simulink model "Katex_FullCar_R2017b_V03"  (R2026a)
settings: Solver=ode1  StopTime=1000  FixedStep=Ts  EnableMultiTasking=on
PostLoadFcn:
  | , if any(exist('dsrtsu_mdlpostloadfcn', 'file') == [2, 3, 6]), try dsrtsu_mdlpostloadfcn('Execute', bdroot); catch fprintf('Error in PostLoadFcn (dsrtsu_mdlpostloadfcn) for model "%s":\n %s\n', bdroot, lasterr); end, end,
  | , if any(exist('dsrtsu_mdlpostloadfcn', 'file') ~= 0), dsrtsu_mdlpostloadfcn('Execute', bdroot); end,
InitFcn:
  | , if any(exist('rtifpga_mdlclblib', 'file') ~= 0), rtifpga_mdlclblib('Init', bdroot); end,
  | 
  | 
  | init
undefined symbols (not defined in the file): locklim_sus, roundN, Ts
libraries: sl_discontinuities x29, simulink_extras x26, simulink x22, mjLib x1
(part 2 of 10)

== system Katex_FullCar_R2017b_V03/Locomotion/Initialization ==
  FLin : Inport
  FRin : Inport  Port=2
  RLin : Inport  Port=3
  RRin : Inport  Port=4
  Bus Creator{1..5} (5 alike) : BusCreator  Inputs=4
  Bus Selector : BusSelector  OutputSignals=FLdrv_velref_mps,FLstr_angref_deg,FLsus_angref_deg
  Bus Selector1 : BusSelector  OutputSignals=FRdrv_velref_mps,FRstr_angref_deg,FRsus_angref_deg
  Bus Selector2 : BusSelector  OutputSignals=RLdrv_velref_mps,RLstr_angref_deg,RLsus_angref_deg
  Bus Selector3 : BusSelector  OutputSignals=RRdrv_velref_mps,RRstr_angref_deg,RRsus_angref_deg
  Subsystem : Subsystem
  Subsystem1 : Subsystem
  Subsystem2 : Subsystem
  Subsystem3 : Subsystem
  Controller : Outport  VectorParamsAs1DForOutWhenUnconnected=off
  tag scope: Controller=global
  wires:
  FLin/1 -> Subsystem/1(In1), Bus Selector/1
  Bus Selector/2 -> Bus Creator4/2  "<FLstr_angref_deg>"
  Bus Selector/3 -> Bus Creator4/3  "<FLsus_angref_deg>"
  Bus Creator4/1 -> Bus Creator5/1  "FL"
  Bus Selector/1 -> Bus Creator4/1  "<FLdrv_velref_mps>"
  FRin/1 -> Subsystem1/1(In1), Bus Selector1/1
  Bus Selector1/1 -> Bus Creator1/1  "<FRdrv_velref_mps>"
  Bus Creator1/1 -> Bus Creator5/2  "FR"
  Bus Creator2/1 -> Bus Creator5/3  "RL"
  RLin/1 -> Subsystem2/1(In1), Bus Selector2/1
  RRin/1 -> Subsystem3/1(In1), Bus Selector3/1
  Bus Creator3/1 -> Bus Creator5/4  "RR"
  Subsystem/1(Out1) -> Bus Creator4/4  "FL_tqctrl"
  Subsystem1/1(Out1) -> Bus Creator1/4  "FR_tqctrl"
  Subsystem2/1(Out1) -> Bus Creator2/4  "RL_tqctrl"
  Subsystem3/1(Out1) -> Bus Creator3/4  "RR_tqctrl"
  Bus Creator5/1 -> [Controller], Controller/1  "Controller"
  Bus Selector1/2 -> Bus Creator1/2  "<FRstr_angref_deg>"
  Bus Selector1/3 -> Bus Creator1/3  "<FRsus_angref_deg>"
  Bus Selector2/1 -> Bus Creator2/1  "<RLdrv_velref_mps>"
  Bus Selector2/2 -> Bus Creator2/2  "<RLstr_angref_deg>"
  Bus Selector2/3 -> Bus Creator2/3  "<RLsus_angref_deg>"
  Bus Selector3/1 -> Bus Creator3/1  "<RRdrv_velref_mps>"
  Bus Selector3/2 -> Bus Creator3/2  "<RRstr_angref_deg>"
  Bus Selector3/3 -> Bus Creator3/3  "<RRsus_angref_deg>"

== system Katex_FullCar_R2017b_V03/MuJoCo Interface/FL_Motor_Control ==
  note: 0: Pos Mode
      | 1: Vel Mode
      | 2: Torque Mode
  In1 : Inport
  Bus Creator1 : BusCreator  Inputs=4
  Constant : Constant  Value=0
  Drv_Driver : Subsystem
  Str_Driver : Subsystem
  Sus_Driver : Subsystem
  Out2 : Outport  VectorParamsAs1DForOutWhenUnconnected=off
  wires:
  [Sus_Driver_Mode] -> Sus_Driver/1(In1)
  In1/1 -> Drv_Driver/2(In2), Str_Driver/2(In2), Sus_Driver/2(In2)
  [Str_Driver_Mode] -> Str_Driver/1(In1)
  [Drv_Driver_Mode] -> Drv_Driver/1(In1)
  Constant/1 -> Bus Creator1/2  "cover_motor"
  Bus Creator1/1 -> Out2/1
  Sus_Driver/1(FL_sus_motor) -> Bus Creator1/1  "FL_sus_act"
  Str_Driver/1(FL_steer_motor) -> Bus Creator1/3  "FL_steer_rev"
  Drv_Driver/1(FL_drive_motor) -> Bus Creator1/4  "FL_drive_act"

== system Katex_FullCar_R2017b_V03/MuJoCo Interface/FR_Motor_Control ==
  note: 0: Pos Mode
      | 1: Vel Mode
      | 2: Torque Mode
  In1 : Inport
  Bus Creator1 : BusCreator  Inputs=4
  Constant : Constant  Value=0
  Drv_Driver : Subsystem
  Str_Driver : Subsystem
  Sus_Driver : Subsystem
  Out2 : Outport  VectorParamsAs1DForOutWhenUnconnected=off
  wires:
  In1/1 -> Sus_Driver/2(In2), Str_Driver/2(In2), Drv_Driver/2(In2)
  Constant/1 -> Bus Creator1/2  "cover_motor"
  Bus Creator1/1 -> Out2/1
  [Sus_Driver_Mode] -> Sus_Driver/1(In1)
  Sus_Driver/1(FR_sus_motor) -> Bus Creator1/1  "FR_sus_act"
  [Str_Driver_Mode] -> Str_Driver/1(In1)
  Str_Driver/1(FR_steer_motor) -> Bus Creator1/3  "FR_steer_rev"
  [Drv_Driver_Mode] -> Drv_Driver/1(In1)
  Drv_Driver/1(FR_drive_motor) -> Bus Creator1/4  "FR_drive_act"

== system Katex_FullCar_R2017b_V03/MuJoCo Interface/RL_Motor_Control ==
  note: 0: Pos Mode
      | 1: Vel Mode
      | 2: Torque Mode
  In1 : Inport
  Bus Creator1 : BusCreator  Inputs=4
  Constant : Constant  Value=0
  Drv_Driver : Subsystem
  Str_Driver : Subsystem
  Sus_Driver : Subsystem
  Out2 : Outport  VectorParamsAs1DForOutWhenUnconnected=off
  wires:
  Bus Creator1/1 -> Out2/1
  Constant/1 -> Bus Creator1/2  "cover_motor"
  In1/1 -> Str_Driver/2(In2), Drv_Driver/2(In2), Sus_Driver/2(In2)
  [Sus_Driver_Mode] -> Sus_Driver/1(In1)
  Sus_Driver/1(RL_sus_motor) -> Bus Creator1/1  "RL_sus_act"
  [Str_Driver_Mode] -> Str_Driver/1(In1)
  Str_Driver/1(RL_steer_motor) -> Bus Creator1/3  "RL_steer_rev"
  [Drv_Driver_Mode] -> Drv_Driver/1(In1)
  Drv_Driver/1(RL_drive_motor) -> Bus Creator1/4  "RL_drive_act"

== system Katex_FullCar_R2017b_V03/MuJoCo Interface/RR_Motor_Control ==
  note: 0: Pos Mode
      | 1: Vel Mode
      | 2: Torque Mode
  In1 : Inport
  Bus Creator1 : BusCreator  Inputs=4
  Constant : Constant  Value=0
  Drv_Driver : Subsystem
  Str_Driver : Subsystem
  Sus_Driver : Subsystem
  Out2 : Outport  VectorParamsAs1DForOutWhenUnconnected=off
  wires:
  In1/1 -> Str_Driver/2(In2), Drv_Driver/2(In2), Sus_Driver/2(In2)
  Constant/1 -> Bus Creator1/2  "cover_motor"
  Bus Creator1/1 -> Out2/1
  [Sus_Driver_Mode] -> Sus_Driver/1(In1)
  Sus_Driver/1(RR_sus_motor) -> Bus Creator1/1  "RR_sus_act"
  [Str_Driver_Mode] -> Str_Driver/1(In1)
  Str_Driver/1(RR_steer_motor) -> Bus Creator1/3  "RR_steer_rev"
  [Drv_Driver_Mode] -> Drv_Driver/1(In1)
  Drv_Driver/1(RR_drive_motor) -> Bus Creator1/4  "RR_drive_act"

== system Katex_FullCar_R2017b_V03/Scope/FL ==
  Plant : Inport
  Controller : Inport  Port=2
  Bus Selector3 : BusSelector  OutputSignals=torque_sensor_FL,ENC_FL_sus,ENC_FL_steer,ENC_FL_drive,Vel_FL_sus,Vel_FL_steer,Vel_FL_drv,FL_sus_actuator_torque
  Bus Selector4 : BusSelector  OutputSignals=FL.FLdrv_velref_mps,FL.FL_tqctrl.FLdrv_tqref_pct,FL.FLstr_angref_deg,FL.FL_tqctrl.FLstr_tqref_pct,FL.FLsus_angref_deg,FL.FL_tqctrl.FLsus_tqref_pct
  Demux : Demux  Outputs=3
  FL_sus_torque : Scope
      settings: ActiveDisplayYMinimum=-1  ActiveDisplayYMaximum=1  DataLoggingVariableName=ScopeData81
  FLdrv_ang[deg] : Scope
      settings: ActiveDisplayYMinimum=-1.4323067935591529  ActiveDisplayYMaximum=1.2660358171832233  DataLoggingVariableName=ScopeData31
  FLdrv_ang[rad] : Scope
      settings: ActiveDisplayYMinimum=-1  ActiveDisplayYMaximum=1  DataLoggingVariableName=ScopeData34
  FLdrv_angvel[rad/s] : Scope
      settings: ActiveDisplayYMinimum=-1  ActiveDisplayYMaximum=1  DataLoggingVariableName=ScopeData68
  FLdrv_torque_x : Scope
      settings: ActiveDisplayYMinimum=-1  ActiveDisplayYMaximum=1  DataLoggingVariableName=ScopeData32
  FLdrv_torque_y : Scope
      settings: ActiveDisplayYMinimum=-1  ActiveDisplayYMaximum=1  DataLoggingVariableName=ScopeData36
  FLdrv_torque_z : Scope
      settings: ActiveDisplayYMinimum=-1  ActiveDisplayYMaximum=1  DataLoggingVariableName=ScopeData29
  FLdrv_tqcmd_pct : Scope
      settings: ActiveDisplayYMinimum=-1  ActiveDisplayYMaximum=1  DataLoggingVariableName=ScopeData33
  FLdrv_tracking_angvel[rad/s] : Scope  NumInputPorts=2
      settings: ActiveDisplayYMinimum=-0.28030249586528166  ActiveDisplayYMaximum=1.28308219274336  DataLoggingVariableName=ScopeData6
  FLdrv_velcmd_mps : Scope
      settings: ActiveDisplayYMinimum=-1  ActiveDisplayYMaximum=1  DataLoggingVariableName=ScopeData35
  FLstr_ang[deg] : Scope
      settings: ActiveDisplayYMinimum=-1  ActiveDisplayYMaximum=1  DataLoggingVariableName=ScopeData22
  FLstr_ang[rad] : Scope
      settings: ActiveDisplayYMinimum=-1  ActiveDisplayYMaximum=1  DataLoggingVariableName=ScopeData38
  FLstr_angcmd_deg : Scope
      settings: ActiveDisplayYMinimum=-1  ActiveDisplayYMaximum=1  DataLoggingVariableName=ScopeData37
  FLstr_angvel[rad/s] : Scope
      settings: ActiveDisplayYMinimum=-1  ActiveDisplayYMaximum=1  DataLoggingVariableName=ScopeData25
  FLstr_tqcmd_pct : Scope
      settings: ActiveDisplayYMinimum=-1  ActiveDisplayYMaximum=1  DataLoggingVariableName=ScopeData40
  FLstr_tracking_ang[deg] : Scope  NumInputPorts=2
      settings: ActiveDisplayYMinimum=-11.551242119792914  ActiveDisplayYMaximum=16.207341064536273
  FLsus_ang[deg] : Scope
      settings: ActiveDisplayYMinimum=-37.299932165417033  ActiveDisplayYMaximum=37.7179622752956  DataLoggingVariableName=ScopeData23
  FLsus_ang[rad] : Scope
      settings: ActiveDisplayYMinimum=-0.24149003314993756  ActiveDisplayYMaximum=2.1734102983494212  DataLoggingVariableName=ScopeData41
  FLsus_angcmd_deg : Scope
      settings: ActiveDisplayYMinimum=-37.5  ActiveDisplayYMaximum=37.5  DataLoggingVariableName=ScopeData42
  FLsus_angvel[rad/s] : Scope
      settings: ActiveDisplayYMinimum=-1  ActiveDisplayYMaximum=1  DataLoggingVariableName=ScopeData24
  FLsus_tqcmd_pct : Scope
      settings: ActiveDisplayYMinimum=-1  ActiveDisplayYMaximum=1  DataLoggingVariableName=ScopeData45
  FLsus_tracking_ang[deg] : Scope  NumInputPorts=2
      settings: ActiveDisplayYMinimum=-59.009615958317596  ActiveDisplayYMaximum=72.033120306985637  DataLoggingVariableName=ScopeData23
  Radians to Degrees : simulink_extras/Transformations/Radians to Degrees
  Radians to Degrees1 : simulink_extras/Transformations/Radians to Degrees
  Radians to Degrees2 : simulink_extras/Transformations/Radians to Degrees
  Subsystem13 : Subsystem
      mask Display: disp('Dri_ref(m/s)_2_motor(rad/s)');
  tag scope: FL_sus_torque=global, FLdrv_ang_deg=global, FLdrv_ang_rad=global, FLdrv_angvel_rads=global, FLstr_ang_deg=global, FLstr_ang_rad=global, FLstr_angvel_rads=global, FLsus_ang_deg=global, FLsus_ang_rad=global, FLsus_angvel_rads=global
  wires:
  Bus Selector4/3 -> FLstr_tracking_ang[deg]/1, FLstr_angcmd_deg/1  "<FLstr_angref_deg>"
  Bus Selector4/2 -> FLdrv_tqcmd_pct/1  "<FLdrv_tqref_pct>"
  Controller/1 -> Bus Selector4/1
  Bus Selector4/5 -> FLsus_tracking_ang[deg]/1, FLsus_angcmd_deg/1  "<FLsus_angref_deg>"
  Bus Selector4/1 -> Subsystem13/1(In1), FLdrv_velcmd_mps/1  "<FLdrv_velref_mps>"
  Bus Selector4/4 -> FLstr_tqcmd_pct/1  "<FLstr_tqref_pct>"
  Bus Selector4/6 -> FLsus_tqcmd_pct/1  "<FLsus_tqref_pct>"
  Plant/1 -> Bus Selector3/1
  Bus Selector3/1 -> Demux/1  "<torque_sensor_FL>"
  Demux/1 -> FLdrv_torque_x/1
  Demux/2 -> FLdrv_torque_y/1
  Demux/3 -> FLdrv_torque_z/1
  Bus Selector3/2 -> [FLsus_ang_rad], Radians to Degrees1/1, FLsus_ang[rad]/1  "<ENC_FL_sus>"
  Bus Selector3/3 -> [FLstr_ang_rad], Radians to Degrees/1, FLstr_ang[rad]/1  "<ENC_FL_steer>"
  Bus Selector3/4 -> [FLdrv_ang_rad], FLdrv_ang[rad]/1, Radians to Degrees2/1  "<ENC_FL_drive>"
  Radians to Degrees/1 -> FLstr_tracking_ang[deg]/2, FLstr_ang[deg]/1, [FLstr_ang_deg]
  Radians to Degrees1/1 -> FLsus_tracking_ang[deg]/2, FLsus_ang[deg]/1, [FLsus_ang_deg]
  Radians to Degrees2/1 -> FLdrv_ang[deg]/1, [FLdrv_ang_deg]
  Bus Selector3/5 -> [FLsus_angvel_rads], FLsus_angvel[rad/s]/1  "<Vel_FL_sus>"
  Bus Selector3/6 -> [FLstr_angvel_rads], FLstr_angvel[rad/s]/1  "<Vel_FL_steer>"
  Bus Selector3/7 -> [FLdrv_angvel_rads], FLdrv_angvel[rad/s]/1  "<Vel_FL_drv>"
  [FLdrv_angvel_rads] -> FLdrv_tracking_angvel[rad/s]/2
  Subsystem13/1(Out1) -> FLdrv_tracking_angvel[rad/s]/1
  Bus Selector3/8 -> FL_sus_torque/1, [FL_sus_torque]  "<FL_sus_actuator_torque>"

== system Katex_FullCar_R2017b_V03/Scope/FR ==
  Plant : Inport
  Controller : Inport  Port=2
  Bus Selector3 : BusSelector  OutputSignals=torque_sensor_FR,ENC_FR_sus,ENC_FR_steer,ENC_FR_drive,Vel_FR_sus,Vel_FR_steer,Vel_FR_drv,FR_sus_actuator_torque
  Bus Selector4 : BusSelector  OutputSignals=FR.FRdrv_velref_mps,FR.FR_tqctrl.FRdrv_tqref_pct,FR.FRstr_angref_deg,FR.FR_tqctrl.FRstr_tqref_pct,FR.FRsus_angref_deg,FR.FR_tqctrl.FRsus_tqref_pct
  Demux : Demux  Outputs=3
  FR_Sus_Torque : Scope
      settings: ActiveDisplayYMinimum=-1  ActiveDisplayYMaximum=1  DataLoggingVariableName=ScopeData93
  FRdrv_ang[deg] : Scope
      settings: ActiveDisplayYMinimum=-1.4323067935591529  ActiveDisplayYMaximum=1.2660358171832233  DataLoggingVariableName=ScopeData26
  FRdrv_ang[rad] : Scope
      settings: ActiveDisplayYMinimum=-0.62767594412282379  ActiveDisplayYMaximum=4.4947333096318136  DataLoggingVariableName=ScopeData30
  FRdrv_angvel[rad/s] : Scope
      settings: ActiveDisplayYMinimum=-1  ActiveDisplayYMaximum=1  DataLoggingVariableName=ScopeData69
  FRdrv_torque_x : Scope
      settings: DataLoggingVariableName=ScopeData39
  FRdrv_torque_y : Scope
      settings: DataLoggingVariableName=ScopeData43
  FRdrv_torque_z : Scope
      settings: DataLoggingVariableName=ScopeData44
  FRdrv_tqcmd_pct : Scope
      settings: DataLoggingVariableName=ScopeData16
  FRdrv_velcmd_mps : Scope
      settings: ActiveDisplayYMinimum=-0.05625  ActiveDisplayYMaximum=0.0062499999999999986  DataLoggingVariableName=ScopeData17
  FRstr_ang[deg] : Scope
      settings: ActiveDisplayYMinimum=-0.68942300067389928  ActiveDisplayYMaximum=1.3010314169983053  DataLoggingVariableName=ScopeData46
  FRstr_ang[rad] : Scope
      settings: ActiveDisplayYMinimum=-1.4323067935591529  ActiveDisplayYMaximum=1.2660358171832233  DataLoggingVariableName=ScopeData47
  FRstr_angcmd_deg : Scope
      settings: ActiveDisplayYMinimum=-1  ActiveDisplayYMaximum=1  DataLoggingVariableName=ScopeData18
  FRstr_angvel[rad/s] : Scope
      settings: ActiveDisplayYMinimum=-1  ActiveDisplayYMaximum=1  DataLoggingVariableName=ScopeData70
  FRstr_tqcmd_pct : Scope
      settings: ActiveDisplayYMinimum=-1  ActiveDisplayYMaximum=1  DataLoggingVariableName=ScopeData19
  FRsus_ang[deg] : Scope
      settings: ActiveDisplayYMinimum=-1.4323067935591529  ActiveDisplayYMaximum=1.2660358171832233  DataLoggingVariableName=ScopeData48
  FRsus_ang[rad] : Scope
      settings: ActiveDisplayYMinimum=-0.24149003314993756  ActiveDisplayYMaximum=2.1734102983494212  DataLoggingVariableName=ScopeData49
  FRsus_angcmd_deg : Scope
      settings: ActiveDisplayYMinimum=-0.15656346548746433  ActiveDisplayYMaximum=1.4090711893871792  DataLoggingVariableName=ScopeData20
  FRsus_angvel[rad/s] : Scope
      settings: ActiveDisplayYMinimum=-1  ActiveDisplayYMaximum=1  DataLoggingVariableName=ScopeData71
  FRsus_tqcmd_pct : Scope
      settings: ActiveDisplayYMinimum=-1  ActiveDisplayYMaximum=1  DataLoggingVariableName=ScopeData21
  Radians to Degrees2 : simulink_extras/Transformations/Radians to Degrees
  Radians to Degrees3 : simulink_extras/Transformations/Radians to Degrees
  Radians to Degrees4 : simulink_extras/Transformations/Radians to Degrees
  tag scope: FR_sus_torque=global, FRdrv_ang_deg=global, FRdrv_ang_rad=global, FRdrv_angvel_rads=global, FRstr_ang_deg=global, FRstr_ang_rad=global, FRstr_angvel_rads=global, FRsus_ang_deg=global, FRsus_ang_rad=global, FRsus_angvel_rads=global
  wires:
  Bus Selector4/3 -> FRstr_angcmd_deg/1  "<FRstr_angref_deg>"
  Bus Selector4/4 -> FRstr_tqcmd_pct/1  "<FRstr_tqref_pct>"
  Bus Selector4/1 -> FRdrv_velcmd_mps/1  "<FRdrv_velref_mps>"
  Bus Selector4/2 -> FRdrv_tqcmd_pct/1  "<FRdrv_tqref_pct>"
  Bus Selector4/5 -> FRsus_angcmd_deg/1  "<FRsus_angref_deg>"
  Bus Selector4/6 -> FRsus_tqcmd_pct/1  "<FRsus_tqref_pct>"
  Demux/2 -> FRdrv_torque_y/1
  Bus Selector3/1 -> Demux/1  "<torque_sensor_FR>"
  Radians to Degrees2/1 -> FRstr_ang[deg]/1, [FRstr_ang_deg]
  Demux/1 -> FRdrv_torque_x/1
  Demux/3 -> FRdrv_torque_z/1
  Bus Selector3/4 -> Radians to Degrees4/1, FRdrv_ang[rad]/1, [FRdrv_ang_rad]  "<ENC_FR_drive>"
  Radians to Degrees4/1 -> FRdrv_ang[deg]/1, [FRdrv_ang_deg]
  Bus Selector3/3 -> Radians to Degrees2/1, FRstr_ang[rad]/1, [FRstr_ang_rad]  "<ENC_FR_steer>"
  Radians to Degrees3/1 -> FRsus_ang[deg]/1, [FRsus_ang_deg]
  Bus Selector3/2 -> [FRsus_ang_rad], Radians to Degrees3/1, FRsus_ang[rad]/1  "<ENC_FR_sus>"
  Controller/1 -> Bus Selector4/1
  Plant/1 -> Bus Selector3/1
  Bus Selector3/6 -> FRstr_angvel[rad/s]/1, [FRstr_angvel_rads]  "<Vel_FR_steer>"
  Bus Selector3/7 -> FRdrv_angvel[rad/s]/1, [FRdrv_angvel_rads]  "<Vel_FR_drv>"
  Bus Selector3/5 -> FRsus_angvel[rad/s]/1, [FRsus_angvel_rads]  "<Vel_FR_sus>"
  Bus Selector3/8 -> [FR_sus_torque], FR_Sus_Torque/1  "<FR_sus_actuator_torque>"

== system Katex_FullCar_R2017b_V03/Scope/IMU ==
  In1 : Inport
  AccX_mps2 : Scope
  AccY_mps2 : Scope
      settings: DataLoggingVariableName=ScopeData2
  AccZ_mps2 : Scope
      settings: DataLoggingVariableName=ScopeData3
  AngPitch_deg : Scope
      settings: ActiveDisplayYMinimum=-1.4665013173998793  ActiveDisplayYMaximum=0.16294459082234145  DataLoggingVariableName=ScopeData8
  AngRoll_deg : Scope
      settings: ActiveDisplayYMinimum=-0.015240922681418762  ActiveDisplayYMaximum=0.083964012205553593  DataLoggingVariableName=ScopeData7
  AngYaw_deg : Scope
      settings: ActiveDisplayYMinimum=-23.87219812859848  ActiveDisplayYMaximum=3.7709983036777981  DataLoggingVariableName=ScopeData15
  Bus Selector : BusSelector  OutputSignals=imu_acc,imu_gyro,trunk_ang
  Demux : Demux  Outputs=3
  Demux1 : Demux  Outputs=3
  Demux2 : Demux  Outputs=3
  Gain1 : Gain
  MATLAB Function : MATLAB Function  TreatAsAtomicUnit=on
  Quaternions to Rotation Angles : Quat2Angle
      settings: AttributesFormatString=Rotation Order: %<rotationOrder>
  Radians to Degrees{,1..5} (6 alike) : simulink_extras/Transformations/Radians to Degrees
  RatePitch_degps : Scope
      settings: DataLoggingVariableName=ScopeData5
  RateRoll_degps : Scope
      settings: DataLoggingVariableName=ScopeData4
  RateYaw_degps : Scope
      settings: DataLoggingVariableName=ScopeData6
  sensor : Gain
  tag scope: AngPitch_deg=global, AngRateYaw_degps=global, AngRoll_deg=global
  wires:
  In1/1 -> Bus Selector/1
  Demux/1 -> AccX_mps2/1
  Demux/2 -> AccY_mps2/1
  Demux/3 -> AccZ_mps2/1
  Bus Selector/1 -> Demux/1  "<imu_acc>"
  Demux1/1 -> Radians to Degrees3/1
  Demux1/2 -> Radians to Degrees4/1
  Demux1/3 -> Radians to Degrees5/1
  Bus Selector/2 -> Demux1/1  "<imu_gyro>"
  Bus Selector/3 -> MATLAB Function/1(q_in)  "<trunk_ang>"
  Quaternions to Rotation Angles/1 -> Demux2/1
  Demux2/2 -> Radians to Degrees1/1
  Demux2/1 -> Radians to Degrees/1
  Demux2/3 -> Radians to Degrees2/1
  Radians to Degrees/1 -> sensor/1
  Radians to Degrees1/1 -> Gain1/1
  Radians to Degrees2/1 -> [AngRoll_deg], AngRoll_deg/1
  Radians to Degrees3/1 -> RateRoll_degps/1
  Radians to Degrees4/1 -> RatePitch_degps/1
  Radians to Degrees5/1 -> [AngRateYaw_degps], RateYaw_degps/1
  MATLAB Function/1(qout) -> Quaternions to Rotation Angles/1
  Gain1/1 -> [AngPitch_deg], AngPitch_deg/1
  sensor/1 -> AngYaw_deg/1  "Sensor"

== system Katex_FullCar_R2017b_V03/Scope/Initialization_Status ==
  InitSta_FLstr : Scope
      settings: ActiveDisplayYMinimum=-1  ActiveDisplayYMaximum=1
  InitSta_FLsus : Scope
      settings: ActiveDisplayYMinimum=-1  ActiveDisplayYMaximum=1  DataLoggingVariableName=ScopeData2
  InitSta_FRstr : Scope
      settings: DataLoggingVariableName=ScopeData8
  InitSta_FRsus : Scope
      settings: DataLoggingVariableName=ScopeData9
  InitSta_RLstr : Scope
      settings: DataLoggingVariableName=ScopeData10
  InitSta_RLsus : Scope
      settings: DataLoggingVariableName=ScopeData11
  InitSta_RRstr : Scope
      settings: DataLoggingVariableName=ScopeData12
  InitSta_RRsus : Scope
      settings: DataLoggingVariableName=ScopeData13
  wires:
  [InitSta_FLstr] -> InitSta_FLstr/1
  [InitSta_FLsus] -> InitSta_FLsus/1
  [InitSta_FRstr] -> InitSta_FRstr/1
  [InitSta_FRsus] -> InitSta_FRsus/1
  [InitSta_RLstr] -> InitSta_RLstr/1
  [InitSta_RLsus] -> InitSta_RLsus/1
  [InitSta_RRstr] -> InitSta_RRstr/1
  [InitSta_RRsus] -> InitSta_RRsus/1

== system Katex_FullCar_R2017b_V03/Scope/RL ==
  Plant : Inport
  Controller : Inport  Port=2
  Bus Selector3 : BusSelector  OutputSignals=torque_sensor_RL,ENC_RL_sus,ENC_RL_steer,ENC_RL_drive,Vel_RL_sus,Vel_RL_steer,Vel_RL_drv,RL_sus_actuator_torque
  Bus Selector4 : BusSelector  OutputSignals=RL.RLdrv_velref_mps,RL.RL_tqctrl.RLdrv_tqref_pct,RL.RLstr_angref_deg,RL.RL_tqctrl.RLstr_tqref_pct,RL.RLsus_angref_deg,RL.RL_tqctrl.RLsus_tqref_pct
  Demux : Demux  Outputs=3
  RL_sus_torque : Scope
      settings: ActiveDisplayYMinimum=-1  ActiveDisplayYMaximum=1  DataLoggingVariableName=ScopeData94
  RLdrv_ang[deg] : Scope
      settings: ActiveDisplayYMinimum=-1.4323067935591529  ActiveDisplayYMaximum=1.2660358171832233  DataLoggingVariableName=ScopeData50
  RLdrv_ang[rad] : Scope
      settings: ActiveDisplayYMinimum=-0.62767594412282379  ActiveDisplayYMaximum=4.4947333096318136  DataLoggingVariableName=ScopeData51
  RLdrv_angvel[rad/s] : Scope
      settings: ActiveDisplayYMinimum=-1  ActiveDisplayYMaximum=1  DataLoggingVariableName=ScopeData72
  RLdrv_torque_x : Scope
      settings: DataLoggingVariableName=ScopeData52
  RLdrv_torque_y : Scope
      settings: DataLoggingVariableName=ScopeData53
  RLdrv_torque_z : Scope
      settings: DataLoggingVariableName=ScopeData54
  RLdrv_tqcmd_pct : Scope
      settings: DataLoggingVariableName=ScopeData33
  RLdrv_velcmd_mps : Scope
      settings: DataLoggingVariableName=ScopeData35
  RLstr_ang[deg] : Scope
      settings: ActiveDisplayYMinimum=-1.4323067935591529  ActiveDisplayYMaximum=1.2660358171832233  DataLoggingVariableName=ScopeData55
  RLstr_ang[rad] : Scope
      settings: ActiveDisplayYMinimum=-1.4323067935591529  ActiveDisplayYMaximum=1.2660358171832233  DataLoggingVariableName=ScopeData56
  RLstr_angcmd_deg : Scope
      settings: DataLoggingVariableName=ScopeData37
  RLstr_angvel[rad/s] : Scope
      settings: ActiveDisplayYMinimum=-1  ActiveDisplayYMaximum=1  DataLoggingVariableName=ScopeData73
  RLstr_tqcmd_pct : Scope
      settings: DataLoggingVariableName=ScopeData40
  RLsus_ang[deg] : Scope
      settings: ActiveDisplayYMinimum=-1.4323067935591529  ActiveDisplayYMaximum=1.2660358171832233  DataLoggingVariableName=ScopeData57
  RLsus_ang[rad] : Scope
      settings: ActiveDisplayYMinimum=-0.24149003314993756  ActiveDisplayYMaximum=2.1734102983494212  DataLoggingVariableName=ScopeData58
  RLsus_angcmd_deg : Scope
      settings: DataLoggingVariableName=ScopeData42
  RLsus_angvel[rad/s] : Scope
      settings: ActiveDisplayYMinimum=-1  ActiveDisplayYMaximum=1  DataLoggingVariableName=ScopeData74
  RLsus_tqcmd_pct : Scope
      settings: DataLoggingVariableName=ScopeData45
  Radians to Degrees2 : simulink_extras/Transformations/Radians to Degrees
  Radians to Degrees3 : simulink_extras/Transformations/Radians to Degrees
  Radians to Degrees4 : simulink_extras/Transformations/Radians to Degrees
  tag scope: RL_sus_torque=global, RLdrv_ang_deg=global, RLdrv_ang_rad=global, RLdrv_angvel_rads=global, RLstr_ang_deg=global, RLstr_ang_rad=global, RLstr_angvel_rads=global, RLsus_ang_deg=global, RLsus_ang_rad=global, RLsus_angvel_rads=global
  wires:
  Bus Selector4/3 -> RLstr_angcmd_deg/1  "<RLstr_angref_deg>"
  Bus Selector4/2 -> RLdrv_tqcmd_pct/1  "<RLdrv_tqref_pct>"
  Controller/1 -> Bus Selector4/1
  Bus Selector4/5 -> RLsus_angcmd_deg/1  "<RLsus_angref_deg>"
  Bus Selector4/1 -> RLdrv_velcmd_mps/1  "<RLdrv_velref_mps>"
  Bus Selector4/4 -> RLstr_tqcmd_pct/1  "<RLstr_tqref_pct>"
  Bus Selector4/6 -> RLsus_tqcmd_pct/1  "<RLsus_tqref_pct>"
  Bus Selector3/1 -> Demux/1  "<torque_sensor_RL>"
  Demux/1 -> RLdrv_torque_x/1
  Radians to Degrees2/1 -> RLstr_ang[deg]/1, [RLstr_ang_deg]
  Radians to Degrees3/1 -> RLsus_ang[deg]/1, [RLsus_ang_deg]
  Bus Selector3/2 -> Radians to Degrees3/1, RLsus_ang[rad]/1, [RLsus_ang_rad]  "<ENC_RL_sus>"
  Radians to Degrees4/1 -> RLdrv_ang[deg]/1, [RLdrv_ang_deg]
  Bus Selector3/4 -> Radians to Degrees4/1, RLdrv_ang[rad]/1, [RLdrv_ang_rad]  "<ENC_RL_drive>"
  Bus Selector3/3 -> Radians to Degrees2/1, RLstr_ang[rad]/1, [RLstr_ang_rad]  "<ENC_RL_steer>"
  Demux/2 -> RLdrv_torque_y/1
  Demux/3 -> RLdrv_torque_z/1
  Plant/1 -> Bus Selector3/1
  Bus Selector3/6 -> RLstr_angvel[rad/s]/1, [RLstr_angvel_rads]  "<Vel_RL_steer>"
  Bus Selector3/7 -> RLdrv_angvel[rad/s]/1, [RLdrv_angvel_rads]  "<Vel_RL_drv>"
  Bus Selector3/5 -> RLsus_angvel[rad/s]/1, [RLsus_angvel_rads]  "<Vel_RL_sus>"
  Bus Selector3/8 -> [RL_sus_torque], RL_sus_torque/1  "<RL_sus_actuator_torque>"

== system Katex_FullCar_R2017b_V03/Scope/RR ==
  Plant : Inport
  Controller : Inport  Port=2
  Bus Selector3 : BusSelector  OutputSignals=torque_sensor_RR,ENC_RR_sus,ENC_RR_steer,ENC_RR_drive,Vel_RR_sus,Vel_RR_steer,Vel_RR_drv,RR_sus_actuator_torque
  Bus Selector4 : BusSelector  OutputSignals=RR.RRdrv_velref_mps,RR.RR_tqctrl.RRdrv_tqref_pct,RR.RRstr_angref_deg,RR.RR_tqctrl.RRstr_tqref_pct,RR.RRsus_angref_deg,RR.RR_tqctrl.RRsus_tqref_pct
  Demux : Demux  Outputs=3
  RLdrv_torque_x : Scope
      settings: DataLoggingVariableName=ScopeData61
  RLdrv_torque_y : Scope
      settings: DataLoggingVariableName=ScopeData62
  RLdrv_torque_z : Scope
      settings: DataLoggingVariableName=ScopeData63
  RR_Sus_torque : Scope
      settings: ActiveDisplayYMinimum=-1  ActiveDisplayYMaximum=1  DataLoggingVariableName=ScopeData95
  RRdrv_ang[deg] : Scope
      settings: ActiveDisplayYMinimum=-1.4323067935591529  ActiveDisplayYMaximum=1.2660358171832233  DataLoggingVariableName=ScopeData59
  RRdrv_ang[rad] : Scope
      settings: ActiveDisplayYMinimum=-0.62767594412282379  ActiveDisplayYMaximum=4.4947333096318136  DataLoggingVariableName=ScopeData60
  RRdrv_angvel[rad/s] : Scope
      settings: ActiveDisplayYMinimum=-1  ActiveDisplayYMaximum=1  DataLoggingVariableName=ScopeData75
  RRdrv_tqcmd_pct : Scope
      settings: DataLoggingVariableName=ScopeData33
  RRdrv_velcmd_mps : Scope
      settings: DataLoggingVariableName=ScopeData35
  RRstr_ang[deg] : Scope
      settings: ActiveDisplayYMinimum=-1.4323067935591529  ActiveDisplayYMaximum=1.2660358171832233  DataLoggingVariableName=ScopeData64
  RRstr_ang[rad] : Scope
      settings: ActiveDisplayYMinimum=-1.4323067935591529  ActiveDisplayYMaximum=1.2660358171832233  DataLoggingVariableName=ScopeData65
  RRstr_angcmd_deg : Scope
      settings: DataLoggingVariableName=ScopeData37
  RRstr_angvel[rad/s] : Scope
      settings: ActiveDisplayYMinimum=-1  ActiveDisplayYMaximum=1  DataLoggingVariableName=ScopeData76
  RRstr_tqcmd_pct : Scope
      settings: DataLoggingVariableName=ScopeData40
  RRsus_ang[deg] : Scope
      settings: ActiveDisplayYMinimum=-1.4323067935591529  ActiveDisplayYMaximum=1.2660358171832233  DataLoggingVariableName=ScopeData66
  RRsus_ang[rad] : Scope
      settings: ActiveDisplayYMinimum=-0.24149003314993756  ActiveDisplayYMaximum=2.1734102983494212  DataLoggingVariableName=ScopeData67
  RRsus_angcmd_deg : Scope
      settings: DataLoggingVariableName=ScopeData42
  RRsus_angvel[rad/s] : Scope
      settings: ActiveDisplayYMinimum=-1  ActiveDisplayYMaximum=1  DataLoggingVariableName=ScopeData77
  RRsus_tqcmd_pct : Scope
      settings: DataLoggingVariableName=ScopeData45
  Radians to Degrees2 : simulink_extras/Transformations/Radians to Degrees
  Radians to Degrees3 : simulink_extras/Transformations/Radians to Degrees
  Radians to Degrees4 : simulink_extras/Transformations/Radians to Degrees
  tag scope: RR_Sus_torque=global, RRdrv_ang_deg=global, RRdrv_ang_rad=global, RRdrv_angvel_rads=global, RRstr_ang_deg=global, RRstr_ang_rad=global, RRstr_angvel_rads=global, RRsus_ang_deg=global, RRsus_ang_rad=global, RRsus_angvel_rads=global
  wires:
  Bus Selector4/3 -> RRstr_angcmd_deg/1  "<RRstr_angref_deg>"
  Bus Selector4/2 -> RRdrv_tqcmd_pct/1  "<RRdrv_tqref_pct>"
  Controller/1 -> Bus Selector4/1
  Bus Selector4/5 -> RRsus_angcmd_deg/1  "<RRsus_angref_deg>"
  Bus Selector4/1 -> RRdrv_velcmd_mps/1  "<RRdrv_velref_mps>"
  Bus Selector4/4 -> RRstr_tqcmd_pct/1  "<RRstr_tqref_pct>"
  Bus Selector4/6 -> RRsus_tqcmd_pct/1  "<RRsus_tqref_pct>"
  Bus Selector3/1 -> Demux/1  "<torque_sensor_RR>"
  Bus Selector3/3 -> Radians to Degrees2/1, RRstr_ang[rad]/1, [RRstr_ang_rad]  "<ENC_RR_steer>"
  Radians to Degrees4/1 -> RRdrv_ang[deg]/1, [RRdrv_ang_deg]
  Demux/3 -> RLdrv_torque_z/1
  Bus Selector3/2 -> Radians to Degrees3/1, RRsus_ang[rad]/1, [RRsus_ang_rad]  "<ENC_RR_sus>"
  Radians to Degrees3/1 -> RRsus_ang[deg]/1, [RRsus_ang_deg]
  Demux/2 -> RLdrv_torque_y/1
  Radians to Degrees2/1 -> RRstr_ang[deg]/1, [RRstr_ang_deg]
  Bus Selector3/4 -> Radians to Degrees4/1, RRdrv_ang[rad]/1, [RRdrv_ang_rad]  "<ENC_RR_drive>"
  Demux/1 -> RLdrv_torque_x/1
  Plant/1 -> Bus Selector3/1
  Bus Selector3/6 -> RRstr_angvel[rad/s]/1, [RRstr_angvel_rads]  "<Vel_RR_steer>"
  Bus Selector3/7 -> RRdrv_angvel[rad/s]/1, [RRdrv_angvel_rads]  "<Vel_RR_drv>"
  Bus Selector3/5 -> RRsus_angvel[rad/s]/1, [RRsus_angvel_rads]  "<Vel_RR_sus>"
  Bus Selector3/8 -> [RR_Sus_torque], RR_Sus_torque/1  "<RR_sus_actuator_torque>"

== system Katex_FullCar_R2017b_V03/Scope/TOUCH ==
  Sensor : Inport
  Bus Selector : BusSelector  OutputSignals=touch_FL,touch_FR,touch_RL,touch_RR
  Compare To Constant{,1..3} (4 alike) : simulink/Logic and Bit Operations/Compare To Constant  relop=>=  const=0.5  OutDataTypeStr=boolean
  FL_Contact_State : Scope
      settings: ActiveDisplayYMinimum=-0.12499999999999997  ActiveDisplayYMaximum=1.125  DataLoggingVariableName=ScopeData89
  FR_Contact_State : Scope
      settings: ActiveDisplayYMinimum=-0.12499999999999997  ActiveDisplayYMaximum=1.125  DataLoggingVariableName=ScopeData90
  RL_Contact_State : Scope
      settings: ActiveDisplayYMinimum=-0.12499999999999997  ActiveDisplayYMaximum=1.125  DataLoggingVariableName=ScopeData91
  RR_Contact_State : Scope
      settings: ActiveDisplayYMinimum=-0.12499999999999997  ActiveDisplayYMaximum=1.125  DataLoggingVariableName=ScopeData92
  wires:
  Sensor/1 -> Bus Selector/1
  Bus Selector/1 -> Compare To Constant/1  "<touch_FL>"
  Compare To Constant/1 -> FL_Contact_State/1
  Compare To Constant1/1 -> FR_Contact_State/1
  Bus Selector/2 -> Compare To Constant1/1  "<touch_FR>"
  Compare To Constant2/1 -> RL_Contact_State/1
  Bus Selector/3 -> Compare To Constant2/1  "<touch_RL>"
  Compare To Constant3/1 -> RR_Contact_State/1
  Bus Selector/4 -> Compare To Constant3/1  "<touch_RR>"

== system Katex_FullCar_R2017b_V03/Scope/Trunk ==
  Sensor : Inport
  Bus Selector : BusSelector  OutputSignals=trunk_vel,trunk_angvel,trunk_pos
  Demux : Demux  Outputs=3
  Demux1 : Demux  Outputs=3
  Demux2 : Demux  Outputs=3
  trunk_angvel_pitch : Scope
      settings: DataLoggingVariableName=ScopeData5
  trunk_angvel_roll : Scope
      settings: DataLoggingVariableName=ScopeData4
  trunk_angvel_yaw : Scope
      settings: DataLoggingVariableName=ScopeData6
  trunk_pos_x : Scope
      settings: DataLoggingVariableName=ScopeData7
  trunk_pos_y : Scope
      settings: DataLoggingVariableName=ScopeData8
  trunk_pos_z : Scope
      settings: DataLoggingVariableName=ScopeData14
  trunk_vel_x : Scope
  trunk_vel_y : Scope
      settings: DataLoggingVariableName=ScopeData2
  trunk_vel_z : Scope
      settings: DataLoggingVariableName=ScopeData3
  wires:
  Sensor/1 -> Bus Selector/1
  Demux/1 -> trunk_vel_x/1
  Demux/2 -> trunk_vel_y/1
  Demux/3 -> trunk_vel_z/1
  Demux1/1 -> trunk_angvel_roll/1
  Demux1/2 -> trunk_angvel_pitch/1
  Demux1/3 -> trunk_angvel_yaw/1
  Demux2/1 -> trunk_pos_x/1
  Demux2/2 -> trunk_pos_y/1
  Bus Selector/1 -> Demux/1  "<trunk_vel>"
  Bus Selector/2 -> Demux1/1  "<trunk_angvel>"
  Bus Selector/3 -> Demux2/1  "<trunk_pos>"
  Demux2/3 -> trunk_pos_z/1

== system Katex_FullCar_R2017b_V03/DGIST/Attitude&Force distribution opt/AX=b, QP ==
  u : Inport
  In2 : Inport  Port=2
  In3 : Inport  Port=3
  In4 : Inport  Port=4
  In5 : Inport  Port=5
  MATLAB Function : MATLAB Function  TreatAsAtomicUnit=on
  Desired Fz [4X1] : Outport
  wires:
  MATLAB Function/1(y) -> Desired Fz [4X1]/1
  u/1 -> MATLAB Function/1(u)
  In2/1 -> MATLAB Function/2(sus_ang_fl)
  In3/1 -> MATLAB Function/3(sus_ang_fr)
  In4/1 -> MATLAB Function/4(sus_ang_rl)
  In5/1 -> MATLAB Function/5(sus_ang_rr)

== system Katex_FullCar_R2017b_V03/DGIST/Attitude&Force distribution opt/Desired Height, Roll, Pitch Caculate ==
  u : Inport
  Roll : Inport  Port=2
  Pitch : Inport  Port=3
  Sus_Ang_FL : Inport  Port=4
  Sus_Ang_FR : Inport  Port=5
  Sus_Ang_RL : Inport  Port=6
  Sus_Ang_RR : Inport  Port=7
  MATLAB Function : MATLAB Function  TreatAsAtomicUnit=on
  Desired Attitude Error [3X1] : Outport
  vx[m/s] : Outport  Port=2
  wires:
  u/1 -> MATLAB Function/1(u)
  Roll/1 -> MATLAB Function/2(roll)
  Pitch/1 -> MATLAB Function/3(pitch)
  Sus_Ang_FL/1 -> MATLAB Function/4(sus_ang_fl)
  Sus_Ang_FR/1 -> MATLAB Function/5(sus_ang_fr)
  Sus_Ang_RL/1 -> MATLAB Function/6(sus_ang_rl)
  Sus_Ang_RR/1 -> MATLAB Function/7(sus_ang_rr)
  MATLAB Function/1(y) -> Desired Attitude Error [3X1]/1  "Desired Attitude error [3X1]"
  MATLAB Function/2(v) -> vx[m/s]/1

== system Katex_FullCar_R2017b_V03/DGIST/Attitude&Force distribution opt/Desired Wrench(PID) ==
  Error : Inport
  Constant : Constant  Value=Ts
  Gain1 : Gain  Gain=-1
  MATLAB Function : MATLAB Function  TreatAsAtomicUnit=on
  Mux{,1..3} (4 alike) : Mux  Inputs=3
  Desired Wrench [3X1] : Outport
  wires:
  Error/1 -> MATLAB Function/1(error)
  MATLAB Function/1(y) -> Desired Wrench [3X1]/1
  Constant/1 -> MATLAB Function/5(Ts)
  [Roll_KP_Gain] -> Mux/2
  [Roll_KI_Gain] -> Mux1/2
  [Roll_KD_Gain] -> Mux2/2
  [Pitch_KD_Gain] -> Mux2/3
  [Pitch_KI_Gain] -> Mux1/3
  [Pitch_KP_Gain] -> Mux/3
  [KD_cutoff] -> MATLAB Function/6(fc)
  [Height_KP_Gain] -> Mux/1
  [Height_KI_Gain] -> Mux1/1
  [Height_KD_Gain] -> Mux2/1
  Mux/1 -> MATLAB Function/2(Kp)
  Mux1/1 -> MATLAB Function/3(Ki)
  Mux2/1 -> MATLAB Function/4(Kd)
  Mux3/1 -> MATLAB Function/8(y_max), Gain1/1
  [PID_height_saturation] -> Mux3/1
  [PID_roll_saturation] -> Mux3/2
  [PID_pitch_saturation] -> Mux3/3
  Gain1/1 -> MATLAB Function/7(y_min)

== system Katex_FullCar_R2017b_V03/DGIST/Attitude&Force distribution opt/GRF to Joint Torque ==
  In1 : Inport
  In2 : Inport  Port=2
  In3 : Inport  Port=3
  In4 : Inport  Port=4
  In5 : Inport  Port=5
  MATLAB Function : MATLAB Function  TreatAsAtomicUnit=on
  Desired_sus_torque[4X1] : Outport
  wires:
  In1/1 -> MATLAB Function/1(u)
  MATLAB Function/1(y) -> Desired_sus_torque[4X1]/1
  In2/1 -> MATLAB Function/2(sus_ang_fl)
  In3/1 -> MATLAB Function/3(sus_ang_fr)
  In4/1 -> MATLAB Function/4(sus_ang_rl)
  In5/1 -> MATLAB Function/5(sus_ang_rr)

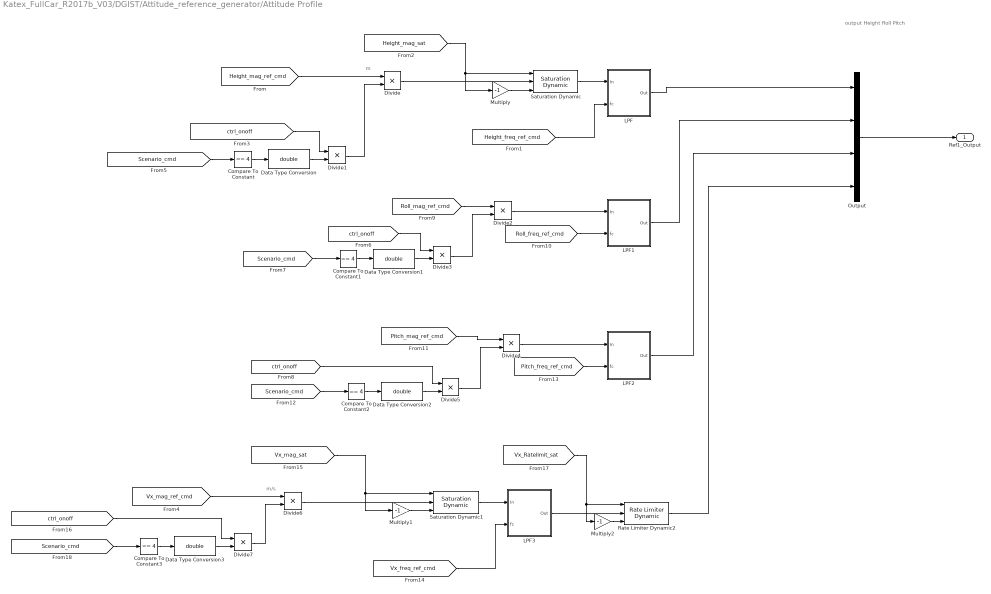
== system Katex_FullCar_R2017b_V03/DGIST/Attitude_reference_generator/Attitude Profile ==
  note: output
      |
      | Height
      | Roll
      | Pitch
  note: m
  note: m/s
  Compare To Constant{,1..3} (4 alike) : simulink/Logic and Bit Operations/Compare To Constant  relop===  const=4  OutDataTypeStr=boolean
  Data Type Conversion{,1..3} (4 alike) : DataTypeConversion  OutDataTypeStr=double  SaturateOnIntegerOverflow=off  RndMeth=Floor
  Divide{,1..7} (8 alike) : Product  Inputs=**
  LPF : Subsystem
  LPF1 : Subsystem
  LPF2 : Subsystem
  LPF3 : Subsystem
  Multiply : Gain  Gain=-1
  Multiply1 : Gain  Gain=-1
  Multiply2 : Gain  Gain=-1
  Output : Mux
  Rate Limiter Dynamic2 : sl_discontinuities/Rate Limiter Dynamic
  Saturation Dynamic : sl_discontinuities/Saturation Dynamic  OutMin=[]  OutMax=[]  OutDataTypeStr=Inherit: Same as second input  OutDataType=fixdt(1, 16)  OutScaling=2^-10  DoSatur=off
  Saturation Dynamic1 : sl_discontinuities/Saturation Dynamic  OutMin=[]  OutMax=[]  OutDataTypeStr=Inherit: Same as second input  OutDataType=fixdt(1, 16)  OutScaling=2^-10  DoSatur=off
  Ref1_Output : Outport
  wires:
  [Pitch_mag_ref_cmd] -> Divide4/1
  [Pitch_freq_ref_cmd] -> LPF2/2(fc)
  Divide4/1 -> LPF2/1(In)
  [Scenario_cmd] -> Compare To Constant2/1
  Divide5/1 -> Divide4/2
  [ctrl_onoff] -> Divide5/1
  Compare To Constant2/1 -> Data Type Conversion2/1
  Data Type Conversion2/1 -> Divide5/2
  [Roll_freq_ref_cmd] -> LPF1/2(fc)
  Divide2/1 -> LPF1/1(In)
  [Roll_mag_ref_cmd] -> Divide2/1
  Divide3/1 -> Divide2/2
  [ctrl_onoff] -> Divide3/1
  Compare To Constant1/1 -> Data Type Conversion1/1
  Data Type Conversion1/1 -> Divide3/2
  [Scenario_cmd] -> Compare To Constant1/1
  Data Type Conversion/1 -> Divide1/2
  Divide1/1 -> Divide/2
  [ctrl_onoff] -> Divide1/1
  Compare To Constant/1 -> Data Type Conversion/1
  [Scenario_cmd] -> Compare To Constant/1
  Multiply/1 -> Saturation Dynamic/3
  [Height_mag_sat] -> Saturation Dynamic/1, Multiply/1
  Output/1 -> Ref1_Output/1
  LPF/1(Out) -> Output/1
  [Height_freq_ref_cmd] -> LPF/2(fc)
  Saturation Dynamic/1 -> LPF/1(In)
  Divide/1 -> Saturation Dynamic/2
  [Height_mag_ref_cmd] -> Divide/1
  LPF1/1(Out) -> Output/2
  LPF2/1(Out) -> Output/3
  [Vx_freq_ref_cmd] -> LPF3/2(fc)
  [Vx_Ratelimit_sat] -> Multiply2/1, Rate Limiter Dynamic2/1
  Multiply1/1 -> Saturation Dynamic1/3
  Divide6/1 -> Saturation Dynamic1/2
  Divide7/1 -> Divide6/2
  Data Type Conversion3/1 -> Divide7/2
  [Vx_mag_sat] -> Multiply1/1, Saturation Dynamic1/1
  LPF3/1(Out) -> Rate Limiter Dynamic2/2
  Compare To Constant3/1 -> Data Type Conversion3/1
  Multiply2/1 -> Rate Limiter Dynamic2/3
  [Scenario_cmd] -> Compare To Constant3/1
  [Vx_mag_ref_cmd] -> Divide6/1
  [ctrl_onoff] -> Divide7/1
  Saturation Dynamic1/1 -> LPF3/1(In)
  Rate Limiter Dynamic2/1 -> Output/4

== system Katex_FullCar_R2017b_V03/DGIST/Subsystem10/LPF ==
  note: LPF : tau = 1/(2*pi*fc)
  note: y(n) = [Ts*{x(n)+x(n-1)}+(2*tau-Ts)*y(n-1)]/(2*tau+Ts)
  note: H(s) = 1/(tau*s+1)
  note: s = 2/Ts*(z-1)/(z+1)
  In : Inport
  fc : Inport  Port=2
  Constant : Constant  Value=Ts  SampleTime=Ts
  Constant1 : Constant  SampleTime=Ts
  Product1 : Product  Inputs=*/  RndMeth=Zero
  Product11 : Product  RndMeth=Zero
  Product2 : Product  Inputs=*/  RndMeth=Zero
  Sum1 : Sum  Inputs=+-  InputSameDT=on  SaturateOnIntegerOverflow=on  OutDataTypeStr=Inherit: Same as first input
  Sum2 : Sum  InputSameDT=on  SaturateOnIntegerOverflow=on  OutDataTypeStr=Inherit: Same as first input
  Sum3 : Sum  InputSameDT=on  SaturateOnIntegerOverflow=on  OutDataTypeStr=Inherit: Same as first input
  Sum4 : Sum  InputSameDT=on  SaturateOnIntegerOverflow=on  OutDataTypeStr=Inherit: Same as first input
  d : UnitDelay  SampleTime=Ts
  d1 : UnitDelay  SampleTime=Ts
  gain : Gain  Gain=Ts  SaturateOnIntegerOverflow=on  OutDataTypeStr=Inherit: Same as input  ParamDataTypeStr=Inherit: Same as input
  gain1 : Gain  Gain=2  SaturateOnIntegerOverflow=on  OutDataTypeStr=Inherit: Same as input  ParamDataTypeStr=Inherit: Same as input
  gain2 : Gain  Gain=2*pi  SaturateOnIntegerOverflow=on  OutDataTypeStr=Inherit: Same as input  ParamDataTypeStr=Inherit: Same as input
  Out : Outport  VectorParamsAs1DForOutWhenUnconnected=off
  wires:
  In/1 -> Sum3/1, d1/1
  d1/1 -> Sum3/2
  Sum3/1 -> gain/1
  gain/1 -> Sum2/1
  Product11/1 -> Sum2/2
  Sum1/1 -> Product11/1
  Constant/1 -> Sum1/2, Sum4/2
  fc/1 -> gain2/1
  gain1/1 -> Sum1/1, Sum4/1
  d/1 -> Product11/2
  Sum2/1 -> Product1/1
  Sum4/1 -> Product1/2
  Product1/1 -> Out/1, d/1
  Product2/1 -> gain1/1
  Constant1/1 -> Product2/1
  gain2/1 -> Product2/2

== system Katex_FullCar_R2017b_V03/DGIST/Subsystem12/LPF ==
  note: LPF : tau = 1/(2*pi*fc)
  note: y(n) = [Ts*{x(n)+x(n-1)}+(2*tau-Ts)*y(n-1)]/(2*tau+Ts)
  note: H(s) = 1/(tau*s+1)
  note: s = 2/Ts*(z-1)/(z+1)
  In : Inport
  fc : Inport  Port=2
  Constant : Constant  Value=Ts  SampleTime=Ts
  Constant1 : Constant  SampleTime=Ts
  Product1 : Product  Inputs=*/  RndMeth=Zero
  Product11 : Product  RndMeth=Zero
  Product2 : Product  Inputs=*/  RndMeth=Zero
  Sum1 : Sum  Inputs=+-  InputSameDT=on  SaturateOnIntegerOverflow=on  OutDataTypeStr=Inherit: Same as first input
  Sum2 : Sum  InputSameDT=on  SaturateOnIntegerOverflow=on  OutDataTypeStr=Inherit: Same as first input
  Sum3 : Sum  InputSameDT=on  SaturateOnIntegerOverflow=on  OutDataTypeStr=Inherit: Same as first input
  Sum4 : Sum  InputSameDT=on  SaturateOnIntegerOverflow=on  OutDataTypeStr=Inherit: Same as first input
  d : UnitDelay  SampleTime=Ts
  d1 : UnitDelay  SampleTime=Ts
  gain : Gain  Gain=Ts  SaturateOnIntegerOverflow=on  OutDataTypeStr=Inherit: Same as input  ParamDataTypeStr=Inherit: Same as input
  gain1 : Gain  Gain=2  SaturateOnIntegerOverflow=on  OutDataTypeStr=Inherit: Same as input  ParamDataTypeStr=Inherit: Same as input
  gain2 : Gain  Gain=2*pi  SaturateOnIntegerOverflow=on  OutDataTypeStr=Inherit: Same as input  ParamDataTypeStr=Inherit: Same as input
  Out : Outport  VectorParamsAs1DForOutWhenUnconnected=off
  wires:
  In/1 -> Sum3/1, d1/1
  d1/1 -> Sum3/2
  Sum3/1 -> gain/1
  gain/1 -> Sum2/1
  Product11/1 -> Sum2/2
  Sum1/1 -> Product11/1
  Constant/1 -> Sum1/2, Sum4/2
  fc/1 -> gain2/1
  gain1/1 -> Sum1/1, Sum4/1
  d/1 -> Product11/2
  Sum2/1 -> Product1/1
  Sum4/1 -> Product1/2
  Product1/1 -> Out/1, d/1
  Product2/1 -> gain1/1
  Constant1/1 -> Product2/1
  gain2/1 -> Product2/2

== system Katex_FullCar_R2017b_V03/DGIST/Subsystem7/LPF ==
  note: LPF : tau = 1/(2*pi*fc)
  note: y(n) = [Ts*{x(n)+x(n-1)}+(2*tau-Ts)*y(n-1)]/(2*tau+Ts)
  note: H(s) = 1/(tau*s+1)
  note: s = 2/Ts*(z-1)/(z+1)
  In : Inport
  fc : Inport  Port=2
  Constant : Constant  Value=Ts  SampleTime=Ts
  Constant1 : Constant  SampleTime=Ts
  Product1 : Product  Inputs=*/  RndMeth=Zero
  Product11 : Product  RndMeth=Zero
  Product2 : Product  Inputs=*/  RndMeth=Zero
  Sum1 : Sum  Inputs=+-  InputSameDT=on  SaturateOnIntegerOverflow=on  OutDataTypeStr=Inherit: Same as first input
  Sum2 : Sum  InputSameDT=on  SaturateOnIntegerOverflow=on  OutDataTypeStr=Inherit: Same as first input
  Sum3 : Sum  InputSameDT=on  SaturateOnIntegerOverflow=on  OutDataTypeStr=Inherit: Same as first input
  Sum4 : Sum  InputSameDT=on  SaturateOnIntegerOverflow=on  OutDataTypeStr=Inherit: Same as first input
  d : UnitDelay  SampleTime=Ts
  d1 : UnitDelay  SampleTime=Ts
  gain : Gain  Gain=Ts  SaturateOnIntegerOverflow=on  OutDataTypeStr=Inherit: Same as input  ParamDataTypeStr=Inherit: Same as input
  gain1 : Gain  Gain=2  SaturateOnIntegerOverflow=on  OutDataTypeStr=Inherit: Same as input  ParamDataTypeStr=Inherit: Same as input
  gain2 : Gain  Gain=2*pi  SaturateOnIntegerOverflow=on  OutDataTypeStr=Inherit: Same as input  ParamDataTypeStr=Inherit: Same as input
  Out : Outport  VectorParamsAs1DForOutWhenUnconnected=off
  wires:
  In/1 -> Sum3/1, d1/1
  d1/1 -> Sum3/2
  Sum3/1 -> gain/1
  gain/1 -> Sum2/1
  Product11/1 -> Sum2/2
  Sum1/1 -> Product11/1
  Constant/1 -> Sum1/2, Sum4/2
  fc/1 -> gain2/1
  gain1/1 -> Sum1/1, Sum4/1
  d/1 -> Product11/2
  Sum2/1 -> Product1/1
  Sum4/1 -> Product1/2
  Product1/1 -> Out/1, d/1
  Product2/1 -> gain1/1
  Constant1/1 -> Product2/1
  gain2/1 -> Product2/2

== system Katex_FullCar_R2017b_V03/DGIST/Subsystem8/LPF ==
  note: LPF : tau = 1/(2*pi*fc)
  note: y(n) = [Ts*{x(n)+x(n-1)}+(2*tau-Ts)*y(n-1)]/(2*tau+Ts)
  note: H(s) = 1/(tau*s+1)
  note: s = 2/Ts*(z-1)/(z+1)
  In : Inport
  fc : Inport  Port=2
  Constant : Constant  Value=Ts  SampleTime=Ts
  Constant1 : Constant  SampleTime=Ts
  Product1 : Product  Inputs=*/  RndMeth=Zero
  Product11 : Product  RndMeth=Zero
  Product2 : Product  Inputs=*/  RndMeth=Zero
  Sum1 : Sum  Inputs=+-  InputSameDT=on  SaturateOnIntegerOverflow=on  OutDataTypeStr=Inherit: Same as first input
  Sum2 : Sum  InputSameDT=on  SaturateOnIntegerOverflow=on  OutDataTypeStr=Inherit: Same as first input
  Sum3 : Sum  InputSameDT=on  SaturateOnIntegerOverflow=on  OutDataTypeStr=Inherit: Same as first input
  Sum4 : Sum  InputSameDT=on  SaturateOnIntegerOverflow=on  OutDataTypeStr=Inherit: Same as first input
  d : UnitDelay  SampleTime=Ts
  d1 : UnitDelay  SampleTime=Ts
  gain : Gain  Gain=Ts  SaturateOnIntegerOverflow=on  OutDataTypeStr=Inherit: Same as input  ParamDataTypeStr=Inherit: Same as input
  gain1 : Gain  Gain=2  SaturateOnIntegerOverflow=on  OutDataTypeStr=Inherit: Same as input  ParamDataTypeStr=Inherit: Same as input
  gain2 : Gain  Gain=2*pi  SaturateOnIntegerOverflow=on  OutDataTypeStr=Inherit: Same as input  ParamDataTypeStr=Inherit: Same as input
  Out : Outport  VectorParamsAs1DForOutWhenUnconnected=off
  wires:
  In/1 -> Sum3/1, d1/1
  d1/1 -> Sum3/2
  Sum3/1 -> gain/1
  gain/1 -> Sum2/1
  Product11/1 -> Sum2/2
  Sum1/1 -> Product11/1
  Constant/1 -> Sum1/2, Sum4/2
  fc/1 -> gain2/1
  gain1/1 -> Sum1/1, Sum4/1
  d/1 -> Product11/2
  Sum2/1 -> Product1/1
  Sum4/1 -> Product1/2
  Product1/1 -> Out/1, d/1
  Product2/1 -> gain1/1
  Constant1/1 -> Product2/1
  gain2/1 -> Product2/2

== system Katex_FullCar_R2017b_V03/DGIST/Subsystem9/LPF ==
  note: LPF : tau = 1/(2*pi*fc)
  note: y(n) = [Ts*{x(n)+x(n-1)}+(2*tau-Ts)*y(n-1)]/(2*tau+Ts)
  note: H(s) = 1/(tau*s+1)
  note: s = 2/Ts*(z-1)/(z+1)
  In : Inport
  fc : Inport  Port=2
  Constant : Constant  Value=Ts  SampleTime=Ts
  Constant1 : Constant  SampleTime=Ts
  Product1 : Product  Inputs=*/  RndMeth=Zero
  Product11 : Product  RndMeth=Zero
  Product2 : Product  Inputs=*/  RndMeth=Zero
  Sum1 : Sum  Inputs=+-  InputSameDT=on  SaturateOnIntegerOverflow=on  OutDataTypeStr=Inherit: Same as first input
  Sum2 : Sum  InputSameDT=on  SaturateOnIntegerOverflow=on  OutDataTypeStr=Inherit: Same as first input
  Sum3 : Sum  InputSameDT=on  SaturateOnIntegerOverflow=on  OutDataTypeStr=Inherit: Same as first input
  Sum4 : Sum  InputSameDT=on  SaturateOnIntegerOverflow=on  OutDataTypeStr=Inherit: Same as first input
  d : UnitDelay  SampleTime=Ts
  d1 : UnitDelay  SampleTime=Ts
  gain : Gain  Gain=Ts  SaturateOnIntegerOverflow=on  OutDataTypeStr=Inherit: Same as input  ParamDataTypeStr=Inherit: Same as input
  gain1 : Gain  Gain=2  SaturateOnIntegerOverflow=on  OutDataTypeStr=Inherit: Same as input  ParamDataTypeStr=Inherit: Same as input
  gain2 : Gain  Gain=2*pi  SaturateOnIntegerOverflow=on  OutDataTypeStr=Inherit: Same as input  ParamDataTypeStr=Inherit: Same as input
  Out : Outport  VectorParamsAs1DForOutWhenUnconnected=off
  wires:
  In/1 -> Sum3/1, d1/1
  d1/1 -> Sum3/2
  Sum3/1 -> gain/1
  gain/1 -> Sum2/1
  Product11/1 -> Sum2/2
  Sum1/1 -> Product11/1
  Constant/1 -> Sum1/2, Sum4/2
  fc/1 -> gain2/1
  gain1/1 -> Sum1/1, Sum4/1
  d/1 -> Product11/2
  Sum2/1 -> Product1/1
  Sum4/1 -> Product1/2
  Product1/1 -> Out/1, d/1
  Product2/1 -> gain1/1
  Constant1/1 -> Product2/1
  gain2/1 -> Product2/2

== system Katex_FullCar_R2017b_V03/DGIST/_High_Level_Ctrl/Chassis_FB_ctrl ==
  note: rad/s
  note: 수정필요
  note: rad/s 여야함
  Abs1 : Abs  Commented=on  SaturateOnIntegerOverflow=off
  Add : Sum  Inputs=+-
  Add1 : Sum  Inputs=+-
  Add2 : Sum
  Add3 : Sum
  Add4 : Sum  Commented=on
  Constant : Constant  Commented=on  Value=2
  Constant1 : Constant  Commented=on  Value=0.1
  Demux : Demux
  Divide : Product  Inputs=**
  Divide1 : Product  Inputs=**
  From3 : From  Commented=on  GotoTag=DriRR_Load_Vel_meas
  From4 : From  Commented=on  GotoTag=DriRR_Load_Vel_meas
  Goto2 : Goto  Commented=on  GotoTag=Avg_vel_meas  TagVisibility=global
  Kinematic_Mapping_FB : MATLAB Function  TreatAsAtomicUnit=on
  Max : MinMax  Commented=on  Function=max  Inputs=2
  Multiply1 : Gain  Gain=180/pi
  Multiply2 : Gain  Gain=pi/180
  Mux : Mux
  Mux1 : Mux  Inputs=2
  P Control : Subsystem
      mask Display: disp('P Control');
  P Control1 : Subsystem
      mask Display: disp('P Control');
  Product : Product  Commented=on  Inputs=*/
  Product1 : Product  Commented=on  Inputs=**
  Slip contro FLl : Subsystem  Commented=on
  Slip control FR : Subsystem  Commented=on
  Subsystem3 : Subsystem  Commented=on
  Vx_Feedback : Constant
  FF_DriveVel_ref : Outport
  FF_SteerPos_ref : Outport  Port=2
  Body_ref_scope : Outport  Port=3
  wires:
  [Vx_FB_ref] -> Kinematic_Mapping_FB/1(Vx_ref)
  [YawRate_FB_ref] -> Kinematic_Mapping_FB/2(YawRate_ref)
  [Steer_Ref_Limit] -> Kinematic_Mapping_FB/6(SteerLimit)
  Kinematic_Mapping_FB/2(SteerPos_ref) -> FF_SteerPos_ref/1
  [Body_Vx_ref] -> Add2/1, Add/1
  Vx_Feedback/1 -> Add/2
  [Body_YawRate_ref] -> Add3/1, Add1/1
  Multiply2/1 -> Add1/2
  P Control/1(Out1) -> Add2/2
  Add2/1 -> [Vx_FB_ref]
  P Control1/1(Out1) -> Add3/2
  Add3/1 -> [YawRate_FB_ref]
  [Wheel_Radius] -> Kinematic_Mapping_FB/5(WheelRadius)
  [Chassis_wheelbase] -> Kinematic_Mapping_FB/3(L)
  [Chassis_wheelTrack] -> Kinematic_Mapping_FB/4(W)
  Add4/1 -> Subsystem3/1(In1), Product/1
  From3/1 -> Add4/1
  Constant/1 -> Product/2
  Constant1/1 -> Max/1
  Product/1 -> Abs1/1
  Abs1/1 -> Max/2
  Max/1 -> Product1/2
  Subsystem3/1(sign) -> Product1/1
  Product1/1 -> Goto2/1
  Kinematic_Mapping_FB/1(DriveVel_ref) -> Demux/1
  Demux/3 -> Mux/3
  Demux/4 -> Mux/4
  Mux/1 -> FF_DriveVel_ref/1
  [Body_Vx_ref] -> Mux1/1
  [Body_YawRate_ref] -> Multiply1/1
  Mux1/1 -> Body_ref_scope/1
  Multiply1/1 -> Mux1/2
  Add/1 -> Divide/1
  Divide/1 -> P Control/1(err)
  [Body_Vx_FB_OnOff] -> Divide/2
  Add1/1 -> Divide1/1
  Divide1/1 -> P Control1/1(err)
  [Body_YawRate_FB_OnOff] -> Divide1/2
  [AngRateYaw_degps] -> Multiply2/1
  From4/1 -> Add4/2
  Demux/1 -> Mux/1
  Demux/2 -> Mux/2
